simulink model "DIPCRT"  (R2015a)
settings: Solver=ode23  SolverMode=SingleTasking  StartTime=0.0  StopTime=3  FixedStep=1e-3  RelTol=1e-3
values from neighbouring files (symbols this model uses):
  deltas = 1000    [DIPCRTinit.m]
  deltav = 5000    [DIPCRTinit.m]
  ds = 1000    [DIPCRTinit.m]
  dv = 5000    [DIPCRTinit.m]
  g = [0;0;0]    [DIPCRTinit.m]
  j0 = 1    [DIPCRTinit.m]
  j1 = 10    [DIPCRTinit.m]
  j2 = 10    [DIPCRTinit.m]
  j3 = 10    [DIPCRTinit.m]
  j4 = 10    [DIPCRTinit.m]
  jv = 1    [DIPCRTinit.m]
  kappas = 2000    [DIPCRTinit.m]
  kappav = 20000    [DIPCRTinit.m]
  kpr = 500    [DIPCRTinit.m]
  kpt = 500    [DIPCRTinit.m]
  ks = 2000    [DIPCRTinit.m]
  kv = 30    [DIPCRTinit.m]
  m0 = 10    [DIPCRTinit.m]
  m1 = 10    [DIPCRTinit.m]
  m2 = 10    [DIPCRTinit.m]
  m3 = 10    [DIPCRTinit.m]
  m4 = 10    [DIPCRTinit.m]
  mv = 10    [DIPCRTinit.m]
libraries: aerolibutil x22, dspinverses x3, aerolibtransform2 x2, simulink x2
(part 1 of 2)
settings Model: CovSFcnEnable=off  Creator=Martin  LastModifiedBy=mangerer
settings OptimizationCC: BlockReduction=off  BooleanDataType=off  OptimizeBlockIOStorage=off  BufferReuse=off  GlobalBufferReuse=off  ExpressionFolding=off  LocalBlockOutputs=off
settings DebuggingCC: SaveWithParameterizedLinksMsg=none  UnderspecifiedInitializationDetection=Classic  MergeDetectMultiDrivingBlocksExec=none  SignalResolutionControl=TryResolveAllWithWarning
settings HardwareCC: TargetUnknown=on

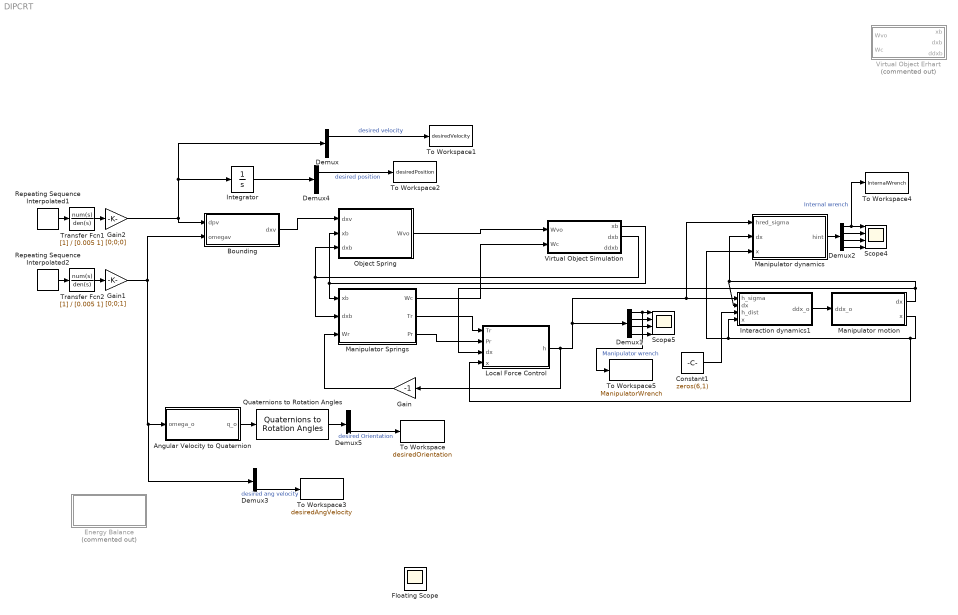
== system DIPCRT ==
  Angular Velocity to Quaternion : Subsystem
  Bounding : Subsystem
  Constant1 : Constant  Value=zeros(6,1)
  Demux{,3..5} (4 alike) : Demux  Outputs=3
  Demux1 : Demux
  Demux2 : Demux
  Energy Balance : Subsystem  Commented=on
  Floating Scope : Scope  NumInputPorts=2
      settings: Floating=on  ShowLegends=on  TimeRange=3  YMin=-0.1~-0.55  YMax=0.05~0.25
  Gain : Gain  Gain=-1
  Gain1 : Gain  Gain=[0;0;1]
  Gain2 : Gain  Gain=[0;0;0]
  Integrator : Integrator
  Interaction dynamics1 : Subsystem
  Local Force Control : Subsystem
  Manipulator Springs : Subsystem
  Manipulator dynamics : Subsystem
  Manipulator motion : Subsystem
  Object Spring : Subsystem
  Quaternions to Rotation Angles : aerolibtransform2/Quaternions to Rotation Angles  rotationOrder=XYZ
  Repeating Sequence Interpolated1 : simulink/Sources/Repeating Sequence Interpolated  OutValues="[0 0 0.225 0 0 0.225 0 0  -0.525 0 0 0.138 0 0].'"  TimeValues=[0 0.1 0.16 0.25 0.9 0.96 1.1 1.8 2 2.2 2.4 2.6 2.8 3].'  LookUpMeth=Interpolation-Use End Values  tsamp=0.001  OutMin=[]  OutMax=[]  OutDataTypeStr=double  OutputDataTypeScalingMode=double  OutDataType=fixdt(0,8)  OutScaling=2^-10
  Repeating Sequence Interpolated2 : simulink/Sources/Repeating Sequence Interpolated  OutValues="[0 0 0.225 0 0 0.225 0 0  -0.525 0 0 0.138 0 0].'"  TimeValues=[0 0.1 0.16 0.25 0.9 0.96 1.1 1.8 2 2.2 2.4 2.6 2.8 3].'  LookUpMeth=Interpolation-Use End Values  tsamp=0.001  OutMin=[]  OutMax=[]  OutDataTypeStr=double  OutputDataTypeScalingMode=double  OutDataType=fixdt(0,8)  OutScaling=2^-10
  Scope4 : Scope  NumInputPorts=4
      settings: ShowLegends=on  YMin=-0.01~-0.01~-0.04~-0.04  YMax=0.04~0.04~0.01~0.01  SaveName=ScopeData6
  Scope5 : Scope  NumInputPorts=4
      settings: ShowLegends=on  TimeRange=3  YMin=-40~-40~-40~-40  YMax=40~40~40~40  SaveName=ScopeData11
  To Workspace : ToWorkspace  VariableName=desiredOrientation  SaveFormat=Timeseries  SampleTime=-1
  To Workspace1 : ToWorkspace  VariableName=desiredVelocity  SaveFormat=Timeseries  SampleTime=-1
  To Workspace2 : ToWorkspace  VariableName=desiredPosition  SaveFormat=Timeseries  SampleTime=-1
  To Workspace3 : ToWorkspace  VariableName=desiredAngVelocity  SaveFormat=Timeseries  SampleTime=-1
  To Workspace4 : ToWorkspace  VariableName=InternalWrench  SaveFormat=Timeseries  SampleTime=-1
  To Workspace5 : ToWorkspace  VariableName=ManipulatorWrench  SaveFormat=Timeseries  SampleTime=-1
  Transfer Fcn1 : TransferFcn  Denominator=[0.005 1]
  Transfer Fcn2 : TransferFcn  Denominator=[0.005 1]
  Virtual Object Erhart : Subsystem  Commented=on
  Virtual Object Simulation : Subsystem
  wires:
  Object Spring/1(Wvo) -> Virtual Object Simulation/1(Wvo)
  Virtual Object Simulation/1(xb) -> Object Spring/2(xb), Manipulator Springs/1(xb)
  Manipulator Springs/1(Wc) -> Virtual Object Simulation/2(Wc)
  Interaction dynamics1/1(ddx_o) -> Manipulator motion/1(ddx_o)
  Constant1/1 -> Interaction dynamics1/3(h_dist)
  Manipulator motion/1(dx) -> Local Force Control/3(dx), Manipulator dynamics/2(dx), Interaction dynamics1/2(dx)
  Manipulator motion/2(x) -> Local Force Control/4(x), Manipulator dynamics/3(x), Interaction dynamics1/4(x)
  Virtual Object Simulation/2(dxb) -> Manipulator Springs/2(dxb), Object Spring/3(dxb)
  Manipulator dynamics/1(hint) -> Demux2/1
  Demux2/2 -> Scope4/2
  Demux2/4 -> Scope4/4
  Demux2/3 -> Scope4/3
  Demux2/1 -> To Workspace4/1, Scope4/1  "Internal wrench"
  Repeating Sequence Interpolated1/1 -> Transfer Fcn1/1
  Transfer Fcn1/1 -> Gain2/1
  Transfer Fcn2/1 -> Gain1/1
  Demux1/2 -> Scope5/2
  Demux1/4 -> Scope5/4
  Demux1/3 -> Scope5/3
  Demux1/1 -> To Workspace5/1, Scope5/1  "Manipulator wrench"
  Quaternions to Rotation Angles/1 -> Demux5/1
  Demux5/3 -> To Workspace/1  "desired Orientation"
  Demux3/3 -> To Workspace3/1  "desired ang velocity"
  Demux4/1 -> To Workspace2/1  "desired position"
  Demux/1 -> To Workspace1/1  "desired velocity"
  Integrator/1 -> Demux4/1
  Angular Velocity to Quaternion/1(q_o) -> Quaternions to Rotation Angles/1
  Gain1/1 -> Demux3/1, Angular Velocity to Quaternion/1(omega_o), Bounding/2(omegav)
  Gain2/1 -> Demux/1, Integrator/1, Bounding/1(dpv)
  Bounding/1(dxv) -> Object Spring/1(dxv)
  Repeating Sequence Interpolated2/1 -> Transfer Fcn2/1
  Manipulator Springs/2(Tr) -> Local Force Control/1(Tr)
  Manipulator Springs/3(Pr) -> Local Force Control/2(Pr)
  Local Force Control/1(h) -> Gain/1, Manipulator dynamics/1(hred_sigma), Interaction dynamics1/1(h_sigma), Demux1/1
  Gain/1 -> Manipulator Springs/3(Wr)

== system DIPCRT/Angular Velocity to Quaternion ==
  omega_o : Inport
  Constant : Constant  Value=0
  Gain : Gain  Gain=0.5
  Integrator : Integrator  InitialCondition=[1; 0; 0; 0]
  Mux : Mux  Inputs=2
  Quaternion Multiplication : aerolibutil/Quaternion Multiplication
  Scope : Scope
      settings: ShowLegends=on  SaveName=ScopeData9
  q_o : Outport
  wires:
  omega_o/1 -> Gain/1
  Gain/1 -> Mux/2
  Constant/1 -> Mux/1
  Quaternion Multiplication/1 -> Integrator/1
  Integrator/1 -> Quaternion Multiplication/2, q_o/1, Scope/1
  Mux/1 -> Quaternion Multiplication/1

== system DIPCRT/Bounding ==
  dpv : Inport
  omegav : Inport  Port=2
  Mux : Mux  Inputs=2
  dxv : Outport
  wires:
  dpv/1 -> Mux/1
  omegav/1 -> Mux/2
  Mux/1 -> dxv/1

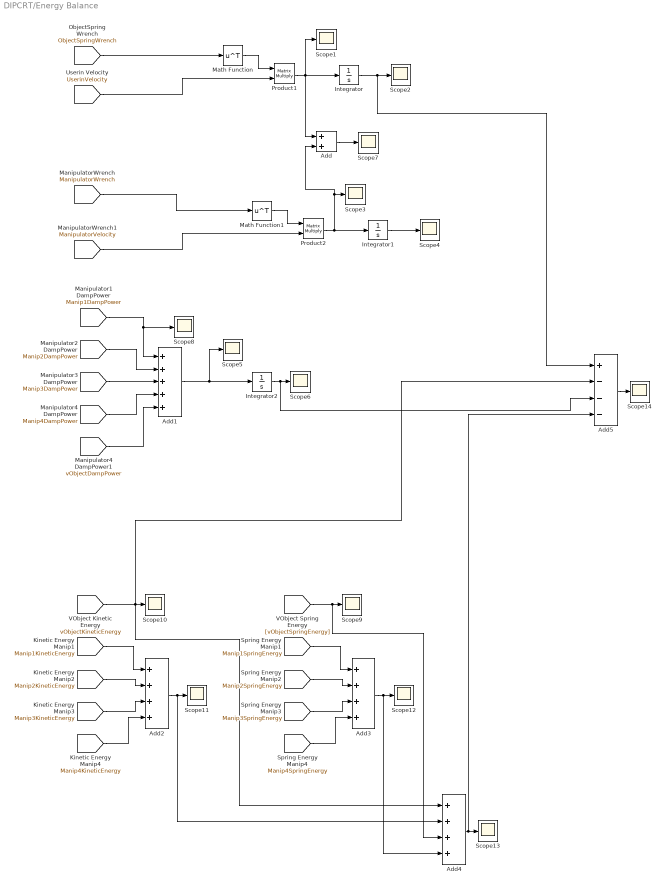
== system DIPCRT/Energy Balance ==
  Add : Sum
  Add1 : Sum  Inputs=+++++
  Add2 : Sum  Inputs=++++
  Add3 : Sum  Inputs=++++
  Add4 : Sum  Inputs=++++
  Add5 : Sum  Inputs=+---
  Integrator : Integrator
  Integrator1 : Integrator
  Integrator2 : Integrator
  Math Function : Math  Operator=transpose  SaturateOnIntegerOverflow=on
  Math Function1 : Math  Operator=transpose  SaturateOnIntegerOverflow=on
  Product1 : Product  Multiplication=Matrix(*)
  Product2 : Product  Multiplication=Matrix(*)
  Scope{1..14} (14 alike) : Scope
      Scope1 settings: YMin=0  YMax=60  SaveName=ScopeData24
      Scope10 settings: YMin=0  YMax=0.08  SaveName=ScopeData29
      Scope11 settings: YMin=0  YMax=12  SaveName=ScopeData30
      Scope12 settings: YMin=0  YMax=0.00021  SaveName=ScopeData31
      Scope13 settings: YMin=0  YMax=50  SaveName=ScopeData32
      Scope14 settings: YMin=102  YMax=108.5  SaveName=ScopeData33
      Scope2 settings: YMin=0  YMax=2100  SaveName=ScopeData18
      Scope3 settings: YMin=-60  YMax=10  SaveName=ScopeData20
      Scope4 settings: YMin=1  YMax=4.5  SaveName=ScopeData21
      Scope5 settings: YMin=-0.3  YMax=0.05  SaveName=ScopeData22
      Scope6 settings: YMin=675  YMax=1000  SaveName=ScopeData25
      Scope7 settings: YMin=-0.3  YMax=0.05  SaveName=ScopeData26
      Scope8 settings: YMin=0  YMax=3e-05  SaveName=ScopeData27
      Scope9 settings: YMin=-4.16334e-17  YMax=0.575  SaveName=ScopeData28
  wires:
  [ObjectSpringWrench] -> Math Function/1
  Product1/1 -> Add/1, Integrator/1, Scope1/1
  Math Function/1 -> Product1/1
  [UserinVelocity] -> Product1/2
  Integrator/1 -> Add5/1, Scope2/1
  Product2/1 -> Integrator1/1, Add/2, Scope3/1
  Math Function1/1 -> Product2/1
  [ManipulatorVelocity] -> Product2/2
  Integrator1/1 -> Scope4/1
  [ManipulatorWrench] -> Math Function1/1
  Add/1 -> Scope7/1
  [Manip1DampPower] -> Scope8/1, Add1/1
  [Manip2DampPower] -> Add1/2
  [Manip3DampPower] -> Add1/3
  [Manip4DampPower] -> Add1/4
  [vObjectDampPower] -> Add1/5
  Add1/1 -> Integrator2/1, Scope5/1
  [vObjectSpringEnergy] -> Add4/3, Scope9/1
  [vObjectKineticEnergy] -> Add5/2, Add4/1, Scope10/1
  [Manip1KineticEnergy] -> Add2/1
  [Manip2KineticEnergy] -> Add2/2
  [Manip3KineticEnergy] -> Add2/3
  [Manip4KineticEnergy] -> Add2/4
  Add2/1 -> Add4/2, Scope11/1
  [Manip1SpringEnergy] -> Add3/1
  [Manip2SpringEnergy] -> Add3/2
  [Manip3SpringEnergy] -> Add3/3
  [Manip4SpringEnergy] -> Add3/4
  Add3/1 -> Add4/4, Scope12/1
  Add4/1 -> Add5/4, Scope13/1
  Integrator2/1 -> Add5/3, Scope6/1
  Add5/1 -> Scope14/1

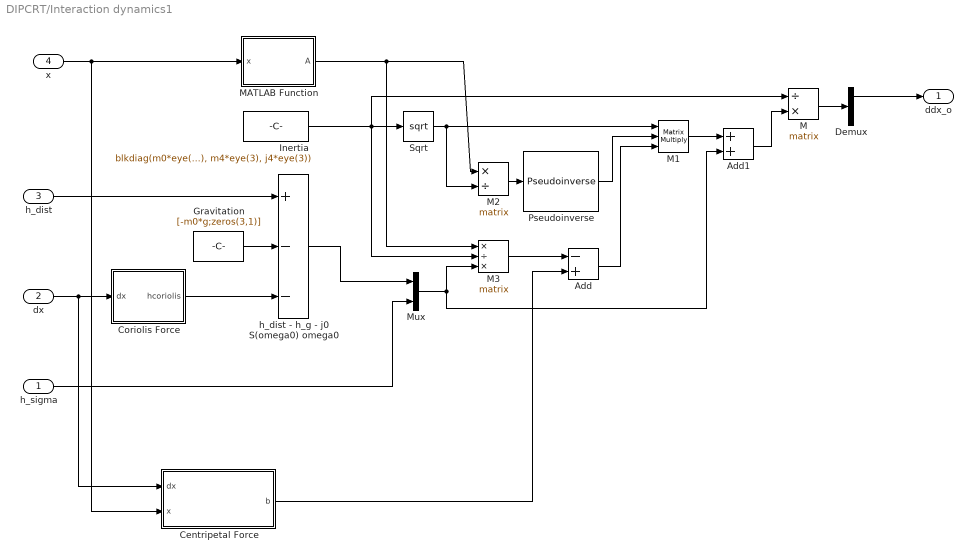
== system DIPCRT/Interaction dynamics1 ==
  h_sigma : Inport
  dx : Inport  Port=2
  h_dist : Inport  Port=3
  x : Inport  Port=4
  Add : Sum  Inputs=-+
  Add1 : Sum
  Centripetal Force : MATLAB Function  TreatAsAtomicUnit=on
  Coriolis Force : MATLAB Function  TreatAsAtomicUnit=on
  Demux : Demux  Outputs=5
  Gravitation : Constant  Value=[-m0*g;zeros(3,1)]
  Inertia : Constant  Value=blkdiag(m0*eye(3),j0*eye(3),m1*eye(3), j1*eye(3), m2*eye(3), j2*eye(3),m3*eye(3), j3*eye(3), m4*eye(3), j4*eye(3))
  M : Product  Inputs=/*  Multiplication=Matrix(*)
  M1 : Product  Inputs=***  Multiplication=Matrix(*)
  M2 : Product  Inputs=*/  Multiplication=Matrix(*)
  M3 : Product  Inputs=*/*  Multiplication=Matrix(*)
  MATLAB Function : MATLAB Function  TreatAsAtomicUnit=on
  Mux : Mux  Inputs=2
  Pseudoinverse : dspinverses/Pseudoinverse  wanterr=off
  Sqrt : Sqrt  SaturateOnIntegerOverflow=on
  "h_dist - h_g - j0 S(omega0) omega0 " : Sum  Inputs=+--
  ddx_o : Outport
  wires:
  h_dist/1 -> "h_dist - h_g - j0 S(omega0) omega0 "/1
  Gravitation/1 -> "h_dist - h_g - j0 S(omega0) omega0 "/2
  dx/1 -> Centripetal Force/1(dx), Coriolis Force/1(dx)
  Coriolis Force/1(hcoriolis) -> "h_dist - h_g - j0 S(omega0) omega0 "/3
  x/1 -> MATLAB Function/1(x), Centripetal Force/2(x)
  Inertia/1 -> M/1, M3/2, Sqrt/1
  Sqrt/1 -> M2/2, M1/1
  MATLAB Function/1(A) -> M3/1, M2/1
  M2/1 -> Pseudoinverse/1
  Pseudoinverse/1 -> M1/2
  Add/1 -> M1/3
  Centripetal Force/1(b) -> Add/2
  M3/1 -> Add/1
  Mux/1 -> Add1/2, M3/3
  "h_dist - h_g - j0 S(omega0) omega0 "/1 -> Mux/1
  h_sigma/1 -> Mux/2
  M/1 -> Demux/1
  Demux/1 -> ddx_o/1
  M1/1 -> Add1/1
  Add1/1 -> M/2

== system DIPCRT/Local Force Control ==
  Tr : Inport
  Pr : Inport  Port=2  PortDimensions=28
  dx : Inport  Port=3
  x : Inport  Port=4
  Add : Sum  Inputs=+++
  Add1 : Sum  Inputs=+-
  Derivative : Derivative
  Manipulator Inertia : Constant  Value=blkdiag(m1*eye(3), j1*eye(3), m2*eye(3), j2*eye(3), m3*eye(3), j3*eye(3), m4*eye(3), j4*eye(3))
  Manipulator kv : Constant  Value=kv*eye(24)
  Product : Product  Multiplication=Matrix(*)
  Product1 : Product  Multiplication=Matrix(*)
  Subsystem : Subsystem
  h : Outport
  wires:
  Product/1 -> h/1
  Manipulator Inertia/1 -> Product/1
  Add/1 -> Product/2
  Tr/1 -> Derivative/1, Add1/1
  dx/1 -> Add1/2
  x/1 -> Subsystem/2(x)
  Subsystem/1(hk) -> Add/1
  Add1/1 -> Product1/2
  Manipulator kv/1 -> Product1/1
  Product1/1 -> Add/2
  Pr/1 -> Subsystem/1(x_r)
  Derivative/1 -> Add/3

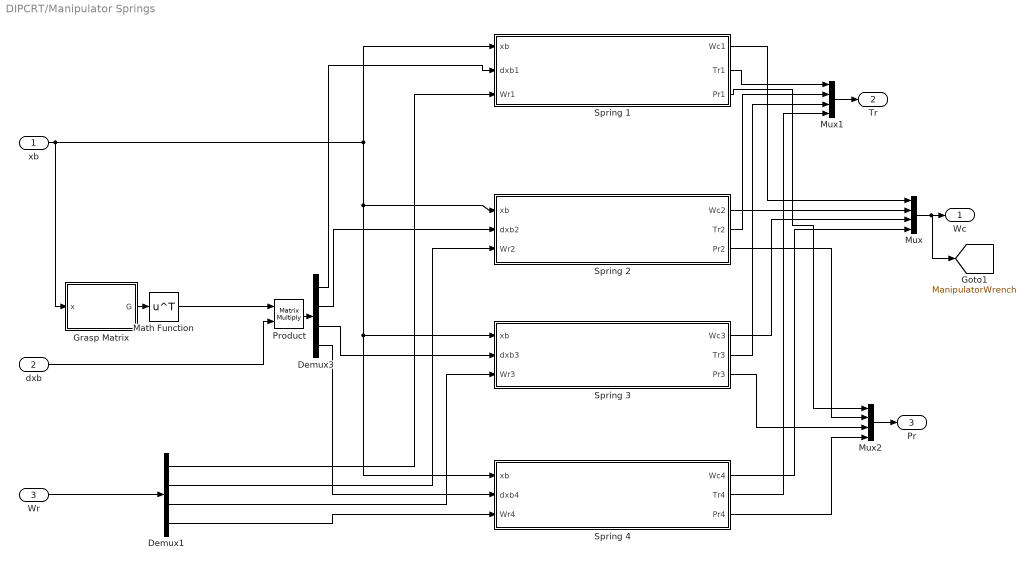
== system DIPCRT/Manipulator Springs ==
  xb : Inport
  dxb : Inport  Port=2
  Wr : Inport  Port=3
  Demux1 : Demux
  Demux3 : Demux
  Grasp Matrix : MATLAB Function  TreatAsAtomicUnit=on
  Math Function : Math  Operator=transpose  SaturateOnIntegerOverflow=on
  Mux : Mux
  Mux1 : Mux
  Mux2 : Mux
  Product : Product  Multiplication=Matrix(*)
  Spring 1 : Subsystem
  Spring 2 : Subsystem
  Spring 3 : Subsystem
  Spring 4 : Subsystem
  Wc : Outport
  Tr : Outport  Port=2
  Pr : Outport  Port=3
  tag scope: ManipulatorWrench=global
  wires:
  Spring 1/1(Wc1) -> Mux/1
  Spring 2/1(Wc2) -> Mux/2
  Mux/1 -> [ManipulatorWrench], Wc/1
  Spring 3/1(Wc3) -> Mux/3
  Spring 4/1(Wc4) -> Mux/4
  Grasp Matrix/1(G) -> Math Function/1
  Math Function/1 -> Product/1
  dxb/1 -> Product/2
  Product/1 -> Demux3/1
  xb/1 -> Spring 1/1(xb), Spring 2/1(xb), Spring 3/1(xb), Spring 4/1(xb), Grasp Matrix/1(x)
  Demux3/1 -> Spring 1/2(dxb1)
  Demux3/2 -> Spring 2/2(dxb2)
  Demux3/3 -> Spring 3/2(dxb3)
  Demux3/4 -> Spring 4/2(dxb4)
  Spring 1/2(Tr1) -> Mux1/1
  Spring 2/2(Tr2) -> Mux1/2
  Spring 3/2(Tr3) -> Mux1/3
  Spring 4/2(Tr4) -> Mux1/4
  Mux1/1 -> Tr/1
  Demux1/4 -> Spring 4/3(Wr4)
  Demux1/3 -> Spring 3/3(Wr3)
  Demux1/2 -> Spring 2/3(Wr2)
  Demux1/1 -> Spring 1/3(Wr1)
  Wr/1 -> Demux1/1
  Mux2/1 -> Pr/1
  Spring 4/3(Pr4) -> Mux2/4
  Spring 3/3(Pr3) -> Mux2/3
  Spring 2/3(Pr2) -> Mux2/2
  Spring 1/3(Pr1) -> Mux2/1

== system DIPCRT/Manipulator dynamics ==
  hred_sigma : Inport
  dx : Inport  Port=2
  x : Inport  Port=3
  A_ * M * A_' : Product  Commented=on  Inputs=*/*  Multiplication=Matrix(*)
  A_'(A_ *M *A_')^-1(b_ - A_/M*hred) : Product  Commented=on  Inputs=*/*  Multiplication=Matrix(*)
  A_/M*hred : Product  Inputs=*/*  Multiplication=Matrix(*)
  Centripal Force : MATLAB Function  TreatAsAtomicUnit=on
  Inertia : Constant  Value=blkdiag(m1*eye(3), j1*eye(3), m2*eye(3), j2*eye(3), m3*eye(3), j3*eye(3), m4*eye(3), j4*eye(3))
  Mult : Product  Inputs=***  Multiplication=Matrix(*)
  Mult1 : Product  Inputs=*/  Multiplication=Matrix(*)
  Pseudoinverse : dspinverses/Pseudoinverse  wanterr=off
  Reduced Constraint Matrix : MATLAB Function  TreatAsAtomicUnit=on
  Sqrt : Sqrt  SaturateOnIntegerOverflow=on
  Transpose : Math  Operator=transpose  SaturateOnIntegerOverflow=on
  World to Object Frame : MATLAB Function  TreatAsAtomicUnit=on
  b_ - A_/M*hred : Sum  Inputs=-+
  hint : Outport
  wires:
  Reduced Constraint Matrix/1(Ared) -> Transpose/1, A_/M*hred/1, Mult1/1
  Inertia/1 -> Sqrt/1, A_/M*hred/2
  dx/1 -> Centripal Force/2(dx)
  A_/M*hred/1 -> b_ - A_/M*hred/1
  hred_sigma/1 -> A_/M*hred/3
  World to Object Frame/1(h_int) -> hint/1
  x/1 -> Centripal Force/1(x), Reduced Constraint Matrix/1(x), World to Object Frame/2(x)
  Centripal Force/1(bred) -> b_ - A_/M*hred/2
  Mult/1 -> World to Object Frame/1(hw)
  b_ - A_/M*hred/1 -> Mult/3
  Sqrt/1 -> Mult1/2, Mult/1
  Mult1/1 -> Pseudoinverse/1
  Pseudoinverse/1 -> Mult/2

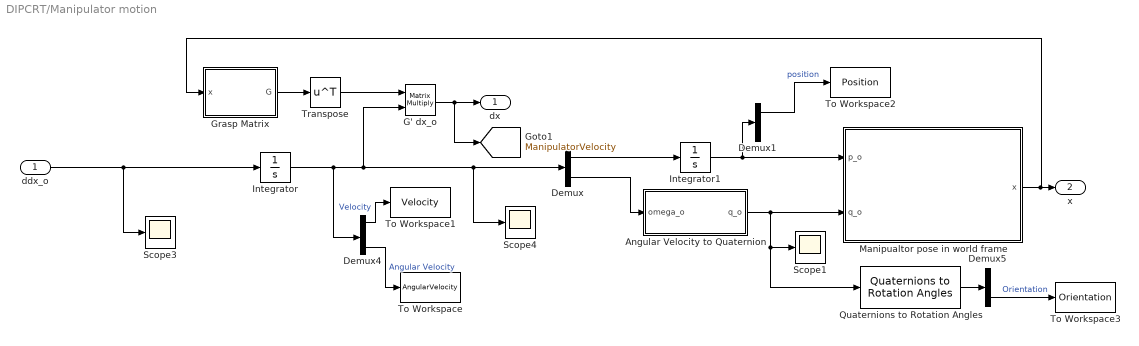
== system DIPCRT/Manipulator motion ==
  ddx_o : Inport
  Angular Velocity to Quaternion : Subsystem
  Demux : Demux  Outputs=2
  Demux1 : Demux  Outputs=3
  Demux4 : Demux  Outputs=6
  Demux5 : Demux  Outputs=3
  G' dx_o : Product  Multiplication=Matrix(*)
  Grasp Matrix : MATLAB Function  TreatAsAtomicUnit=on
  Integrator : Integrator  InitialCondition=zeros(6,1)
  Integrator1 : Integrator  InitialCondition=[0 0 0]'
  Manipualtor pose in world frame : MATLAB Function  TreatAsAtomicUnit=on
  Quaternions to Rotation Angles : aerolibtransform2/Quaternions to Rotation Angles  rotationOrder=XYZ
  Scope1 : Scope
      settings: SaveName=ScopeData13
  Scope3 : Scope
      settings: SaveName=ScopeData7
  Scope4 : Scope
      settings: SaveName=ScopeData16
  To Workspace : ToWorkspace  VariableName=AngularVelocity  SaveFormat=Timeseries  SampleTime=-1
  To Workspace1 : ToWorkspace  VariableName=Velocity  SaveFormat=Timeseries  SampleTime=-1
  To Workspace2 : ToWorkspace  VariableName=Position  SaveFormat=Timeseries  SampleTime=-1
  To Workspace3 : ToWorkspace  VariableName=Orientation  SaveFormat=Timeseries  SampleTime=-1
  Transpose : Math  Operator=transpose  SaturateOnIntegerOverflow=on
  dx : Outport
  x : Outport  Port=2
  tag scope: ManipulatorVelocity=global
  wires:
  ddx_o/1 -> Scope3/1, Integrator/1
  Integrator/1 -> Demux4/1, G' dx_o/2, Scope4/1, Demux/1
  Grasp Matrix/1(G) -> Transpose/1
  Transpose/1 -> G' dx_o/1
  G' dx_o/1 -> [ManipulatorVelocity], dx/1
  Demux/2 -> Angular Velocity to Quaternion/1(omega_o)
  Demux/1 -> Integrator1/1
  Integrator1/1 -> Demux1/1, Manipualtor pose in world frame/1(p_o)
  Manipualtor pose in world frame/1(x) -> Grasp Matrix/1(x), x/1
  Angular Velocity to Quaternion/1(q_o) -> Scope1/1, Quaternions to Rotation Angles/1, Manipualtor pose in world frame/2(q_o)
  Demux4/1 -> To Workspace1/1  "Velocity"
  Demux4/6 -> To Workspace/1  "Angular Velocity"
  Quaternions to Rotation Angles/1 -> Demux5/1
  Demux5/3 -> To Workspace3/1  "Orientation"
  Demux1/1 -> To Workspace2/1  "position"

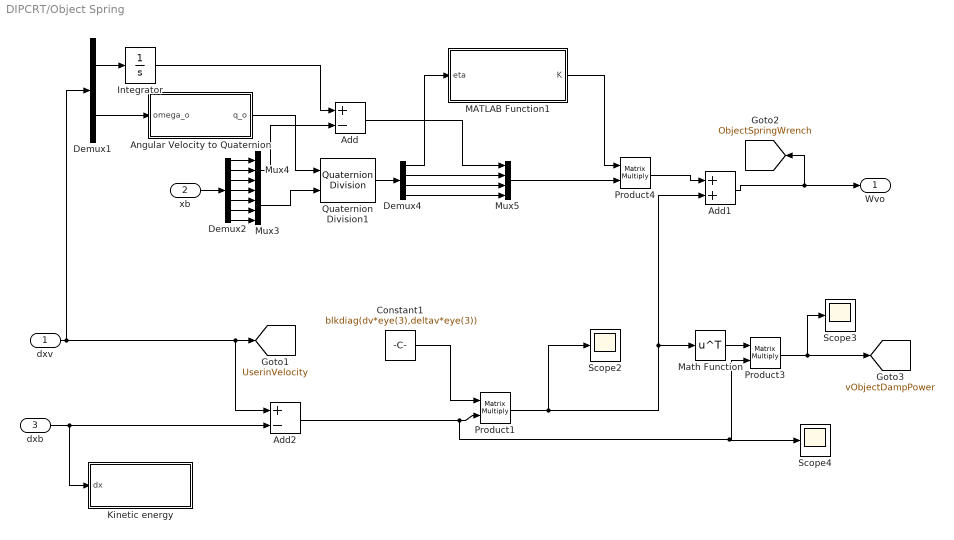
== system DIPCRT/Object Spring ==
  dxv : Inport
  xb : Inport  Port=2
  dxb : Inport  Port=3
  Add : Sum  Inputs=+-
  Add1 : Sum
  Add2 : Sum  Inputs=+-
  Angular Velocity to Quaternion : Subsystem
  Constant1 : Constant  Value=blkdiag(dv*eye(3),deltav*eye(3))
  Demux1 : Demux  Outputs=2
  Demux2 : Demux  Outputs=7
  Demux4 : Demux
  Integrator : Integrator
  Kinetic energy : Subsystem
  MATLAB Function1 : MATLAB Function  TreatAsAtomicUnit=on
  Math Function : Math  Operator=transpose  SaturateOnIntegerOverflow=on
  Mux3 : Mux
  Mux4 : Mux  Inputs=3
  Mux5 : Mux
  Product1 : Product  Multiplication=Matrix(*)
  Product3 : Product  Multiplication=Matrix(*)
  Product4 : Product  Multiplication=Matrix(*)
  Quaternion Division1 : aerolibutil/Quaternion Division
  Scope2 : Scope
      settings: YMin=-1500  YMax=6500  SaveName=ScopeData4
  Scope3 : Scope
      settings: YMin=0  YMax=8500  SaveName=ScopeData2
  Scope4 : Scope
      settings: YMin=-3.5  YMax=3  SaveName=ScopeData35
  Wvo : Outport
  tag scope: ObjectSpringWrench=global, UserinVelocity=global, vObjectDampPower=global
  wires:
  Add1/1 -> [ObjectSpringWrench], Wvo/1
  Product4/1 -> Add1/1
  Product1/1 -> Scope2/1, Math Function/1, Add1/2
  MATLAB Function1/1(K) -> Product4/1
  Demux4/1 -> MATLAB Function1/1(eta)
  Add/1 -> Mux5/1
  Demux4/2 -> Mux5/2
  Demux4/3 -> Mux5/3
  Demux4/4 -> Mux5/4
  Quaternion Division1/1 -> Demux4/1
  xb/1 -> Demux2/1
  Demux2/4 -> Mux3/1
  Demux2/5 -> Mux3/2
  Demux2/6 -> Mux3/3
  Demux2/7 -> Mux3/4
  Demux2/1 -> Mux4/1
  Demux2/2 -> Mux4/2
  Demux2/3 -> Mux4/3
  Mux4/1 -> Add/2
  Mux3/1 -> Quaternion Division1/2
  Add2/1 -> Scope4/1, Product3/2, Product1/2
  dxv/1 -> Demux1/1, [UserinVelocity], Add2/1
  dxb/1 -> Kinetic energy/1(dx), Add2/2
  Product3/1 -> Scope3/1, [vObjectDampPower]
  Math Function/1 -> Product3/1
  Mux5/1 -> Product4/2
  Demux1/1 -> Integrator/1
  Integrator/1 -> Add/1
  Demux1/2 -> Angular Velocity to Quaternion/1(omega_o)
  Angular Velocity to Quaternion/1(q_o) -> Quaternion Division1/1
  Constant1/1 -> Product1/1

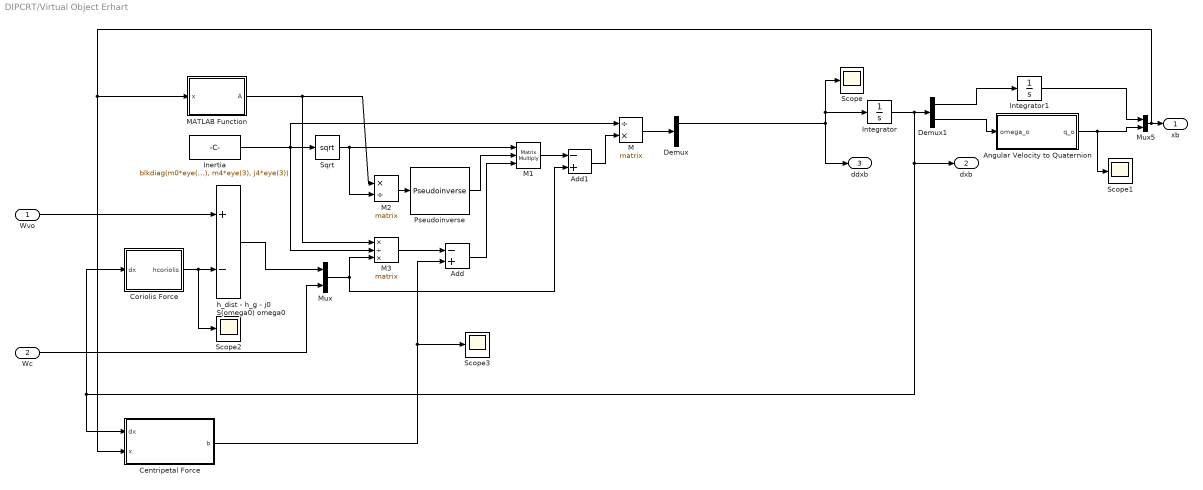
== system DIPCRT/Virtual Object Erhart ==
  Wvo : Inport
  Wc : Inport  Port=2
  Add : Sum  Inputs=-+
  Add1 : Sum  Inputs=-+
  Angular Velocity to Quaternion : Subsystem
  Centripetal Force : MATLAB Function  TreatAsAtomicUnit=on
  Coriolis Force : MATLAB Function  TreatAsAtomicUnit=on
  Demux : Demux  Outputs=5
  Demux1 : Demux  Outputs=2
  Inertia : Constant  Value=blkdiag(m0*eye(3),j0*eye(3),m1*eye(3), j1*eye(3), m2*eye(3), j2*eye(3),m3*eye(3), j3*eye(3), m4*eye(3), j4*eye(3))
  Integrator : Integrator  InitialCondition=zeros(6,1)
  Integrator1 : Integrator  InitialCondition=[0 0 0]'
  M : Product  Inputs=/*  Multiplication=Matrix(*)
  M1 : Product  Inputs=***  Multiplication=Matrix(*)
  M2 : Product  Inputs=*/  Multiplication=Matrix(*)
  M3 : Product  Inputs=*/*  Multiplication=Matrix(*)
  MATLAB Function : MATLAB Function  TreatAsAtomicUnit=on
  Mux : Mux  Inputs=2
  Mux5 : Mux  Inputs=2
  Pseudoinverse : dspinverses/Pseudoinverse  wanterr=off
  Scope{,1..3} (4 alike) : Scope
      Scope1 settings: SaveName=ScopeData8
      Scope2 settings: SaveName=ScopeData15
      Scope3 settings: YMin=-1  YMax=1  SaveName=ScopeData17
  Sqrt : Sqrt  SaturateOnIntegerOverflow=on
  "h_dist - h_g - j0 S(omega0) omega0 " : Sum  Inputs=+-
  xb : Outport
  dxb : Outport  Port=2
  ddxb : Outport  Port=3
  wires:
  Demux/1 -> Scope/1, Integrator/1, ddxb/1
  Integrator/1 -> Demux1/1, Coriolis Force/1(dx), Centripetal Force/1(dx), dxb/1
  Demux1/2 -> Angular Velocity to Quaternion/1(omega_o)
  Demux1/1 -> Integrator1/1
  Integrator1/1 -> Mux5/1
  Angular Velocity to Quaternion/1(q_o) -> Scope1/1, Mux5/2
  Wvo/1 -> "h_dist - h_g - j0 S(omega0) omega0 "/1
  Coriolis Force/1(hcoriolis) -> Scope2/1, "h_dist - h_g - j0 S(omega0) omega0 "/2
  Mux5/1 -> MATLAB Function/1(x), Centripetal Force/2(x), xb/1
  Inertia/1 -> M/1, M3/2, Sqrt/1
  Sqrt/1 -> M2/2, M1/1
  MATLAB Function/1(A) -> M3/1, M2/1
  M2/1 -> Pseudoinverse/1
  Pseudoinverse/1 -> M1/2
  Add/1 -> M1/3
  Centripetal Force/1(b) -> Scope3/1, Add/2
  M3/1 -> Add/1
  Mux/1 -> Add1/2, M3/3
  "h_dist - h_g - j0 S(omega0) omega0 "/1 -> Mux/1
  Wc/1 -> Mux/2
  M1/1 -> Add1/1
  Add1/1 -> M/2
  M/1 -> Demux/1

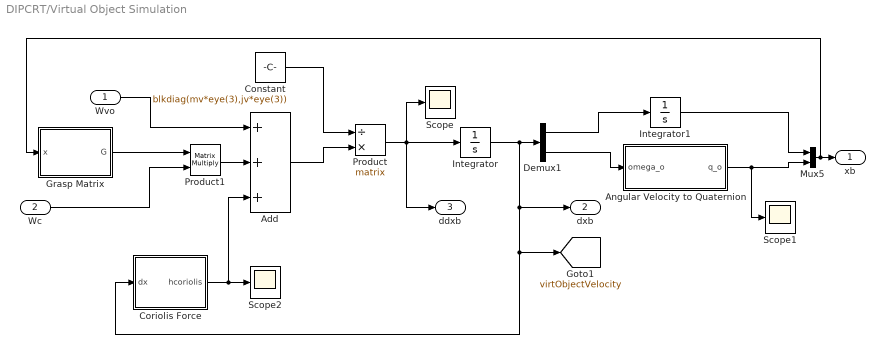
== system DIPCRT/Virtual Object Simulation ==
  Wvo : Inport
  Wc : Inport  Port=2
  Add : Sum  Inputs=+++
  Angular Velocity to Quaternion : Subsystem
  Constant : Constant  Value=blkdiag(mv*eye(3),jv*eye(3))
  Coriolis Force : MATLAB Function  TreatAsAtomicUnit=on
  Demux1 : Demux  Outputs=2
  Grasp Matrix : MATLAB Function  TreatAsAtomicUnit=on
  Integrator : Integrator  InitialCondition=zeros(6,1)
  Integrator1 : Integrator  InitialCondition=[0 0 0]'
  Mux5 : Mux  Inputs=2
  Product : Product  Inputs=/*  Multiplication=Matrix(*)
  Product1 : Product  Inputs=**  Multiplication=Matrix(*)
  Scope : Scope
  Scope1 : Scope
      settings: SaveName=ScopeData8
  Scope2 : Scope
      settings: YMin=-0.008  YMax=0.008  SaveName=ScopeData10
  xb : Outport
  dxb : Outport  Port=2
  ddxb : Outport  Port=3
  tag scope: virtObjectVelocity=global
  wires:
  Add/1 -> Product/2
  Constant/1 -> Product/1
  Product/1 -> ddxb/1, Scope/1, Integrator/1
  Integrator/1 -> Demux1/1, [virtObjectVelocity], Coriolis Force/1(dx), dxb/1
  Demux1/2 -> Angular Velocity to Quaternion/1(omega_o)
  Demux1/1 -> Integrator1/1
  Integrator1/1 -> Mux5/1
  Angular Velocity to Quaternion/1(q_o) -> Scope1/1, Mux5/2
  Mux5/1 -> Grasp Matrix/1(x), xb/1
  Wvo/1 -> Add/1
  Product1/1 -> Add/2
  Grasp Matrix/1(G) -> Product1/1
  Wc/1 -> Product1/2
  Coriolis Force/1(hcoriolis) -> Scope2/1, Add/3

== system DIPCRT/Local Force Control/Subsystem ==
  x_r : Inport
  x : Inport  Port=2
  Demux : Demux
  Demux1 : Demux
  Mux : Mux
  Subsystem : Subsystem
  Subsystem1 : Subsystem
  Subsystem2 : Subsystem
  Subsystem3 : Subsystem
  hk : Outport
  wires:
  x_r/1 -> Demux/1
  x/1 -> Demux1/1
  Demux/1 -> Subsystem/1(x_r1)
  Demux/2 -> Subsystem1/1(x_r2)
  Demux/3 -> Subsystem2/1(x_r3)
  Demux/4 -> Subsystem3/1(x_r4)
  Demux1/1 -> Subsystem/2(x1)
  Demux1/2 -> Subsystem1/2(x2)
  Demux1/3 -> Subsystem2/2(x3)
  Demux1/4 -> Subsystem3/2(x4)
  Subsystem/1(hk1) -> Mux/1
  Subsystem1/1(hk2) -> Mux/2
  Subsystem2/1(hk3) -> Mux/3
  Subsystem3/1(hk4) -> Mux/4
  Mux/1 -> hk/1

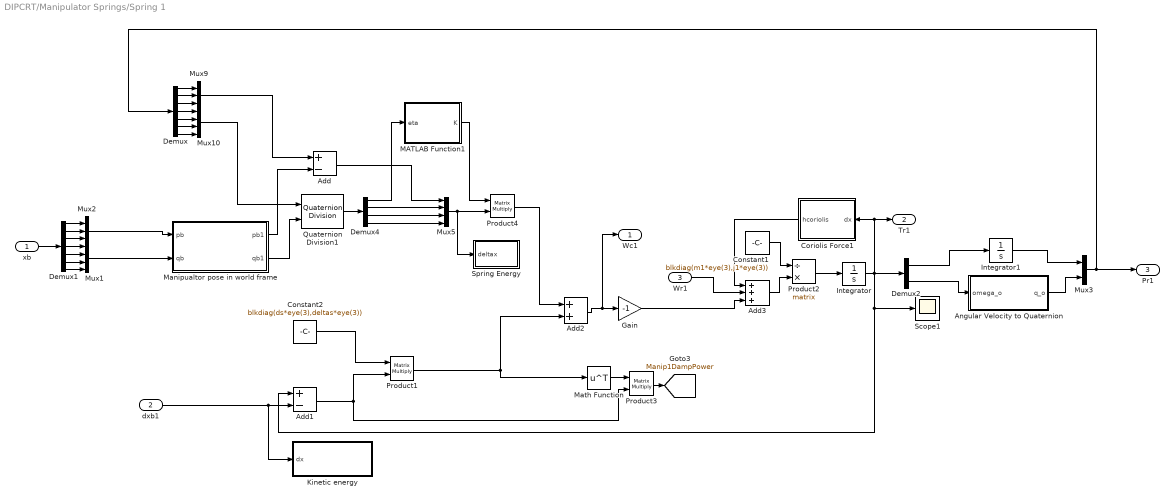
== system DIPCRT/Manipulator Springs/Spring 1 ==
  xb : Inport
  dxb1 : Inport  Port=2
  Wr1 : Inport  Port=3
  Add : Sum  Inputs=+-
  Add1 : Sum  Inputs=+-
  Add2 : Sum
  Add3 : Sum  Inputs=+++
  Angular Velocity to Quaternion : Subsystem
  Constant1 : Constant  Value=blkdiag(m1*eye(3),j1*eye(3))
  Constant2 : Constant  Value=blkdiag(ds*eye(3),deltas*eye(3))
  Coriolis Force1 : MATLAB Function  TreatAsAtomicUnit=on
  Demux : Demux  Outputs=7
  Demux1 : Demux  Outputs=7
  Demux2 : Demux  Outputs=2
  Demux4 : Demux
  Gain : Gain  Gain=-1
  Integrator : Integrator  InitialCondition=zeros(6,1)
  Integrator1 : Integrator  InitialCondition=[1 0 0]'
  Kinetic energy : Subsystem
  MATLAB Function1 : MATLAB Function  TreatAsAtomicUnit=on
  Manipualtor pose in world frame : MATLAB Function  TreatAsAtomicUnit=on
  Math Function : Math  Operator=transpose  SaturateOnIntegerOverflow=on
  Mux1 : Mux
  Mux10 : Mux
  Mux2 : Mux  Inputs=3
  Mux3 : Mux  Inputs=2
  Mux5 : Mux
  Mux9 : Mux  Inputs=3
  Product1 : Product  Multiplication=Matrix(*)
  Product2 : Product  Inputs=/*  Multiplication=Matrix(*)
  Product3 : Product  Multiplication=Matrix(*)
  Product4 : Product  Multiplication=Matrix(*)
  Quaternion Division1 : aerolibutil/Quaternion Division
  Scope1 : Scope
      settings: YMin=-1.5  YMax=0.5  SaveName=ScopeData38
  Spring Energy : Subsystem
  Wc1 : Outport
  Tr1 : Outport  Port=2
  Pr1 : Outport  Port=3  PortDimensions=7
  tag scope: Manip1DampPower=global
  wires:
  Constant2/1 -> Product1/1
  Add2/1 -> Gain/1, Wc1/1
  Demux/1 -> Mux9/1
  Demux/2 -> Mux9/2
  Demux/3 -> Mux9/3
  Demux/4 -> Mux10/1
  Demux/5 -> Mux10/2
  Demux/6 -> Mux10/3
  Demux/7 -> Mux10/4
  MATLAB Function1/1(K) -> Product4/1
  Demux4/1 -> MATLAB Function1/1(eta)
  Add/1 -> Mux5/1
  Demux4/2 -> Mux5/2
  Demux4/3 -> Mux5/3
  Demux4/4 -> Mux5/4
  Quaternion Division1/1 -> Demux4/1
  Mux5/1 -> Spring Energy/1(deltax), Product4/2
  Mux9/1 -> Add/1
  Manipualtor pose in world frame/1(pb1) -> Add/2
  Product4/1 -> Add2/1
  Mux10/1 -> Quaternion Division1/1
  Manipualtor pose in world frame/2(qb1) -> Quaternion Division1/2
  Add1/1 -> Product1/2, Product3/2
  dxb1/1 -> Kinetic energy/1(dx), Add1/2
  Demux1/1 -> Mux2/1
  Demux1/2 -> Mux2/2
  Demux1/3 -> Mux2/3
  Demux1/4 -> Mux1/1
  Demux1/5 -> Mux1/2
  Demux1/6 -> Mux1/3
  Demux1/7 -> Mux1/4
  Mux2/1 -> Manipualtor pose in world frame/1(pb)
  Mux1/1 -> Manipualtor pose in world frame/2(qb)
  xb/1 -> Demux1/1
  Product1/1 -> Add2/2, Math Function/1
  Math Function/1 -> Product3/1
  Product3/1 -> [Manip1DampPower]
  Product2/1 -> Integrator/1
  Add3/1 -> Product2/2
  Coriolis Force1/1(hcoriolis) -> Add3/1
  Demux2/2 -> Angular Velocity to Quaternion/1(omega_o)
  Demux2/1 -> Integrator1/1
  Gain/1 -> Add3/3
  Constant1/1 -> Product2/1
  Wr1/1 -> Add3/2
  Integrator/1 -> Demux2/1, Coriolis Force1/1(dx), Tr1/1, Add1/1, Scope1/1
  Angular Velocity to Quaternion/1(q_o) -> Mux3/2
  Integrator1/1 -> Mux3/1
  Mux3/1 -> Pr1/1, Demux/1

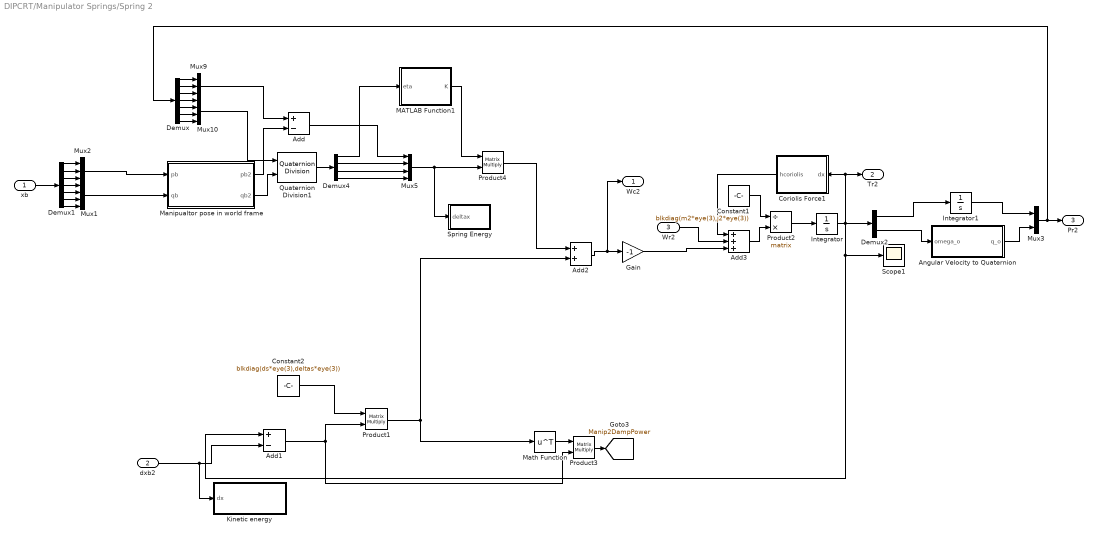
== system DIPCRT/Manipulator Springs/Spring 2 ==
  xb : Inport
  dxb2 : Inport  Port=2
  Wr2 : Inport  Port=3
  Add : Sum  Inputs=+-
  Add1 : Sum  Inputs=+-
  Add2 : Sum
  Add3 : Sum  Inputs=+++
  Angular Velocity to Quaternion : Subsystem
  Constant1 : Constant  Value=blkdiag(m2*eye(3),j2*eye(3))
  Constant2 : Constant  Value=blkdiag(ds*eye(3),deltas*eye(3))
  Coriolis Force1 : MATLAB Function  TreatAsAtomicUnit=on
  Demux : Demux  Outputs=7
  Demux1 : Demux  Outputs=7
  Demux2 : Demux  Outputs=2
  Demux4 : Demux
  Gain : Gain  Gain=-1
  Integrator : Integrator  InitialCondition=zeros(6,1)
  Integrator1 : Integrator  InitialCondition=[0 1 0]'
  Kinetic energy : Subsystem
  MATLAB Function1 : MATLAB Function  TreatAsAtomicUnit=on
  Manipualtor pose in world frame : MATLAB Function  TreatAsAtomicUnit=on
  Math Function : Math  Operator=transpose  SaturateOnIntegerOverflow=on
  Mux1 : Mux
  Mux10 : Mux
  Mux2 : Mux  Inputs=3
  Mux3 : Mux  Inputs=2
  Mux5 : Mux
  Mux9 : Mux  Inputs=3
  Product1 : Product  Multiplication=Matrix(*)
  Product2 : Product  Inputs=/*  Multiplication=Matrix(*)
  Product3 : Product  Multiplication=Matrix(*)
  Product4 : Product  Multiplication=Matrix(*)
  Quaternion Division1 : aerolibutil/Quaternion Division
  Scope1 : Scope
      settings: SaveName=ScopeData3
  Spring Energy : Subsystem
  Wc2 : Outport
  Tr2 : Outport  Port=2
  Pr2 : Outport  Port=3  PortDimensions=7
  tag scope: Manip2DampPower=global
  wires:
  Constant2/1 -> Product1/1
  Demux/1 -> Mux9/1
  Demux/2 -> Mux9/2
  Demux/3 -> Mux9/3
  Demux/4 -> Mux10/1
  Demux/5 -> Mux10/2
  Demux/6 -> Mux10/3
  Demux/7 -> Mux10/4
  MATLAB Function1/1(K) -> Product4/1
  Demux4/1 -> MATLAB Function1/1(eta)
  Add/1 -> Mux5/1
  Demux4/2 -> Mux5/2
  Demux4/3 -> Mux5/3
  Demux4/4 -> Mux5/4
  Quaternion Division1/1 -> Demux4/1
  Mux5/1 -> Spring Energy/1(deltax), Product4/2
  Mux9/1 -> Add/1
  Manipualtor pose in world frame/1(pb2) -> Add/2
  Manipualtor pose in world frame/2(qb2) -> Quaternion Division1/2
  Mux10/1 -> Quaternion Division1/1
  Add2/1 -> Wc2/1, Gain/1
  Product4/1 -> Add2/1
  dxb2/1 -> Kinetic energy/1(dx), Add1/2
  xb/1 -> Demux1/1
  Demux1/1 -> Mux2/1
  Demux1/2 -> Mux2/2
  Demux1/3 -> Mux2/3
  Demux1/4 -> Mux1/1
  Demux1/5 -> Mux1/2
  Demux1/6 -> Mux1/3
  Demux1/7 -> Mux1/4
  Mux2/1 -> Manipualtor pose in world frame/1(pb)
  Mux1/1 -> Manipualtor pose in world frame/2(qb)
  Add1/1 -> Product1/2, Product3/2
  Product1/1 -> Add2/2, Math Function/1
  Math Function/1 -> Product3/1
  Product3/1 -> [Manip2DampPower]
  Product2/1 -> Integrator/1
  Add3/1 -> Product2/2
  Coriolis Force1/1(hcoriolis) -> Add3/1
  Demux2/2 -> Angular Velocity to Quaternion/1(omega_o)
  Demux2/1 -> Integrator1/1
  Constant1/1 -> Product2/1
  Wr2/1 -> Add3/2
  Integrator/1 -> Demux2/1, Coriolis Force1/1(dx), Tr2/1, Add1/1, Scope1/1
  Angular Velocity to Quaternion/1(q_o) -> Mux3/2
  Integrator1/1 -> Mux3/1
  Gain/1 -> Add3/3
  Mux3/1 -> Pr2/1, Demux/1

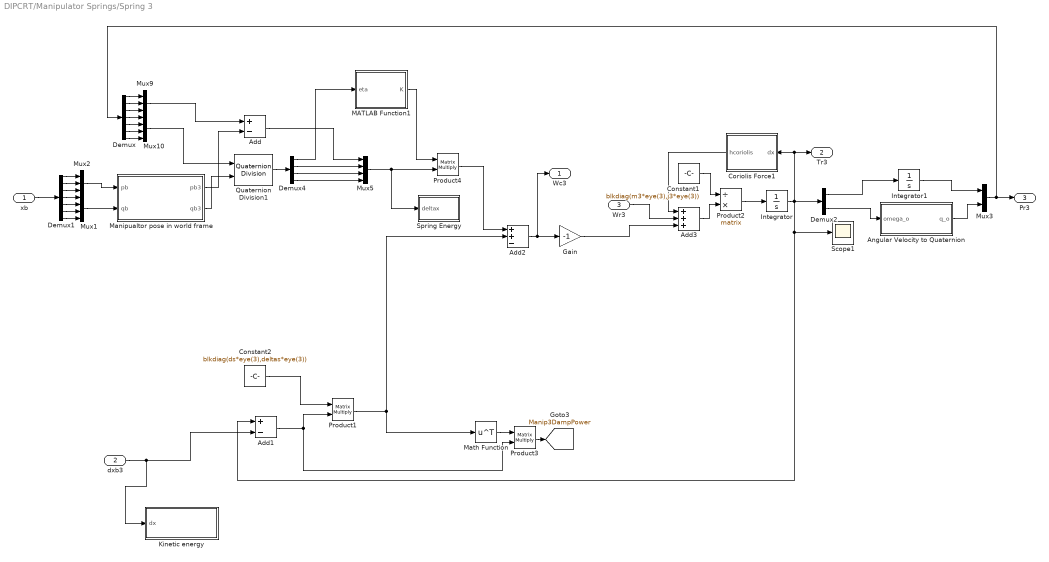
== system DIPCRT/Manipulator Springs/Spring 3 ==
  xb : Inport
  dxb3 : Inport  Port=2
  Wr3 : Inport  Port=3
  Add : Sum  Inputs=+-
  Add1 : Sum  Inputs=+-
  Add2 : Sum  Inputs=++-
  Add3 : Sum  Inputs=+++
  Angular Velocity to Quaternion : Subsystem
  Constant1 : Constant  Value=blkdiag(m3*eye(3),j3*eye(3))
  Constant2 : Constant  Value=blkdiag(ds*eye(3),deltas*eye(3))
  Coriolis Force1 : MATLAB Function  TreatAsAtomicUnit=on
  Demux : Demux  Outputs=7
  Demux1 : Demux  Outputs=7
  Demux2 : Demux  Outputs=2
  Demux4 : Demux
  Gain : Gain  Gain=-1
  Integrator : Integrator  InitialCondition=zeros(6,1)
  Integrator1 : Integrator  InitialCondition=[-1 0 0]'
  Kinetic energy : Subsystem
  MATLAB Function1 : MATLAB Function  TreatAsAtomicUnit=on
  Manipualtor pose in world frame : MATLAB Function  TreatAsAtomicUnit=on
  Math Function : Math  Operator=transpose  SaturateOnIntegerOverflow=on
  Mux1 : Mux
  Mux10 : Mux
  Mux2 : Mux  Inputs=3
  Mux3 : Mux  Inputs=2
  Mux5 : Mux
  Mux9 : Mux  Inputs=3
  Product1 : Product  Multiplication=Matrix(*)
  Product2 : Product  Inputs=/*  Multiplication=Matrix(*)
  Product3 : Product  Multiplication=Matrix(*)
  Product4 : Product  Multiplication=Matrix(*)
  Quaternion Division1 : aerolibutil/Quaternion Division
  Scope1 : Scope
      settings: SaveName=ScopeData36
  Spring Energy : Subsystem
  Wc3 : Outport
  Tr3 : Outport  Port=2
  Pr3 : Outport  Port=3  PortDimensions=7
  tag scope: Manip3DampPower=global
  wires:
  Constant2/1 -> Product1/1
  Add2/1 -> Gain/1, Wc3/1
  Demux/1 -> Mux9/1
  Demux/2 -> Mux9/2
  Demux/3 -> Mux9/3
  Demux/4 -> Mux10/1
  Demux/5 -> Mux10/2
  Demux/6 -> Mux10/3
  Demux/7 -> Mux10/4
  MATLAB Function1/1(K) -> Product4/1
  Demux4/1 -> MATLAB Function1/1(eta)
  Add/1 -> Mux5/1
  Demux4/2 -> Mux5/2
  Demux4/3 -> Mux5/3
  Demux4/4 -> Mux5/4
  Quaternion Division1/1 -> Demux4/1
  Mux5/1 -> Spring Energy/1(deltax), Product4/2
  Product4/1 -> Add2/1
  Mux9/1 -> Add/1
  Manipualtor pose in world frame/1(pb3) -> Add/2
  Mux10/1 -> Quaternion Division1/1
  Manipualtor pose in world frame/2(qb3) -> Quaternion Division1/2
  dxb3/1 -> Add1/2, Kinetic energy/1(dx)
  xb/1 -> Demux1/1
  Demux1/1 -> Mux2/1
  Demux1/2 -> Mux2/2
  Demux1/3 -> Mux2/3
  Demux1/4 -> Mux1/1
  Demux1/5 -> Mux1/2
  Demux1/6 -> Mux1/3
  Demux1/7 -> Mux1/4
  Mux2/1 -> Manipualtor pose in world frame/1(pb)
  Mux1/1 -> Manipualtor pose in world frame/2(qb)
  Add1/1 -> Product1/2, Product3/2
  Product1/1 -> Add2/2, Math Function/1
  Math Function/1 -> Product3/1
  Product3/1 -> [Manip3DampPower]
  Product2/1 -> Integrator/1
  Add3/1 -> Product2/2
  Coriolis Force1/1(hcoriolis) -> Add3/1
  Demux2/2 -> Angular Velocity to Quaternion/1(omega_o)
  Demux2/1 -> Integrator1/1
  Constant1/1 -> Product2/1
  Wr3/1 -> Add3/2
  Integrator/1 -> Demux2/1, Coriolis Force1/1(dx), Tr3/1, Add1/1, Scope1/1
  Angular Velocity to Quaternion/1(q_o) -> Mux3/2
  Integrator1/1 -> Mux3/1
  Gain/1 -> Add3/3
  Mux3/1 -> Pr3/1, Demux/1

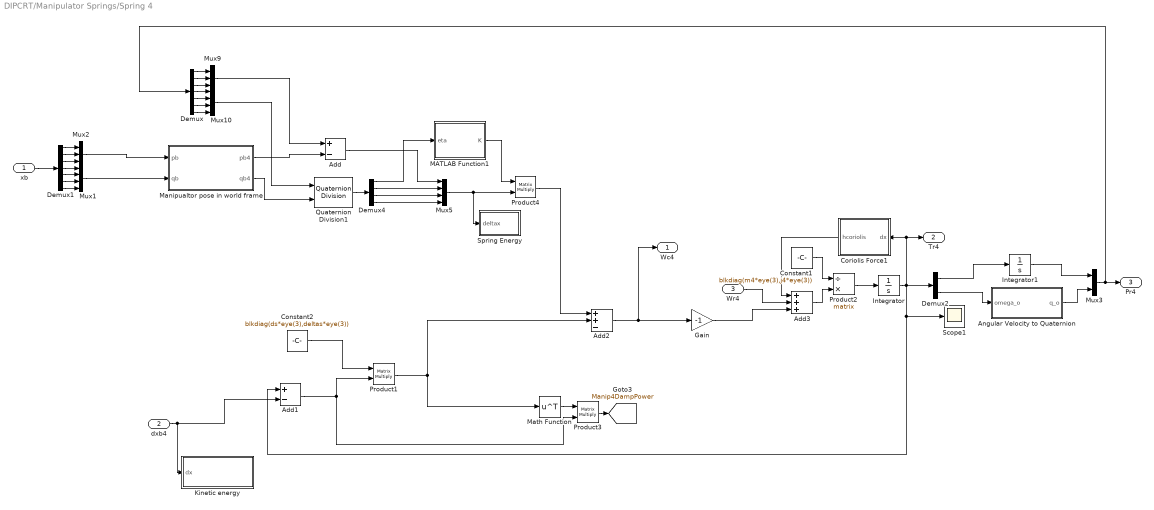
== system DIPCRT/Manipulator Springs/Spring 4 ==
  xb : Inport
  dxb4 : Inport  Port=2
  Wr4 : Inport  Port=3
  Add : Sum  Inputs=+-
  Add1 : Sum  Inputs=+-
  Add2 : Sum  Inputs=++-
  Add3 : Sum  Inputs=+++
  Angular Velocity to Quaternion : Subsystem
  Constant1 : Constant  Value=blkdiag(m4*eye(3),j4*eye(3))
  Constant2 : Constant  Value=blkdiag(ds*eye(3),deltas*eye(3))
  Coriolis Force1 : MATLAB Function  TreatAsAtomicUnit=on
  Demux : Demux  Outputs=7
  Demux1 : Demux  Outputs=7
  Demux2 : Demux  Outputs=2
  Demux4 : Demux
  Gain : Gain  Gain=-1
  Integrator : Integrator  InitialCondition=zeros(6,1)
  Integrator1 : Integrator  InitialCondition=[0 -1 0]'
  Kinetic energy : Subsystem
  MATLAB Function1 : MATLAB Function  TreatAsAtomicUnit=on
  Manipualtor pose in world frame : MATLAB Function  TreatAsAtomicUnit=on
  Math Function : Math  Operator=transpose  SaturateOnIntegerOverflow=on
  Mux1 : Mux
  Mux10 : Mux
  Mux2 : Mux  Inputs=3
  Mux3 : Mux  Inputs=2
  Mux5 : Mux
  Mux9 : Mux  Inputs=3
  Product1 : Product  Multiplication=Matrix(*)
  Product2 : Product  Inputs=/*  Multiplication=Matrix(*)
  Product3 : Product  Multiplication=Matrix(*)
  Product4 : Product  Multiplication=Matrix(*)
  Quaternion Division1 : aerolibutil/Quaternion Division
  Scope1 : Scope
      settings: SaveName=ScopeData37
  Spring Energy : Subsystem
  Wc4 : Outport
  Tr4 : Outport  Port=2
  Pr4 : Outport  Port=3  PortDimensions=7
  tag scope: Manip4DampPower=global
  wires:
  Constant2/1 -> Product1/1
  Add2/1 -> Gain/1, Wc4/1
  Demux/1 -> Mux9/1
  Demux/2 -> Mux9/2
  Demux/3 -> Mux9/3
  Demux/4 -> Mux10/1
  Demux/5 -> Mux10/2
  Demux/6 -> Mux10/3
  Demux/7 -> Mux10/4
  Demux4/2 -> Mux5/2
  Demux4/3 -> Mux5/3
  Demux4/4 -> Mux5/4
  Quaternion Division1/1 -> Demux4/1
  Mux5/1 -> Spring Energy/1(deltax), Product4/2
  MATLAB Function1/1(K) -> Product4/1
  Demux4/1 -> MATLAB Function1/1(eta)
  Add/1 -> Mux5/1
  Mux9/1 -> Add/1
  Manipualtor pose in world frame/1(pb4) -> Add/2
  Mux10/1 -> Quaternion Division1/1
  Manipualtor pose in world frame/2(qb4) -> Quaternion Division1/2
  Product4/1 -> Add2/1
  dxb4/1 -> Kinetic energy/1(dx), Add1/2
  xb/1 -> Demux1/1
  Demux1/1 -> Mux2/1
  Demux1/2 -> Mux2/2
  Demux1/3 -> Mux2/3
  Demux1/4 -> Mux1/1
  Demux1/5 -> Mux1/2
  Demux1/6 -> Mux1/3
  Demux1/7 -> Mux1/4
  Mux2/1 -> Manipualtor pose in world frame/1(pb)
  Mux1/1 -> Manipualtor pose in world frame/2(qb)
  Add1/1 -> Product1/2, Product3/2
  Product1/1 -> Add2/2, Math Function/1
  Math Function/1 -> Product3/1
  Product3/1 -> [Manip4DampPower]
  Product2/1 -> Integrator/1
  Add3/1 -> Product2/2
  Coriolis Force1/1(hcoriolis) -> Add3/1
  Demux2/2 -> Angular Velocity to Quaternion/1(omega_o)
  Demux2/1 -> Integrator1/1
  Constant1/1 -> Product2/1
  Wr4/1 -> Add3/2
  Integrator/1 -> Demux2/1, Coriolis Force1/1(dx), Tr4/1, Add1/1, Scope1/1
  Angular Velocity to Quaternion/1(q_o) -> Mux3/2
  Integrator1/1 -> Mux3/1
  Gain/1 -> Add3/3
  Mux3/1 -> Pr4/1, Demux/1

== system DIPCRT/Manipulator motion/Angular Velocity to Quaternion ==
  omega_o : Inport
  Constant : Constant  Value=0
  Gain : Gain  Gain=0.5
  Integrator : Integrator  InitialCondition=[1; 0; 0; 0]
  Mux : Mux  Inputs=2
  Quaternion Multiplication : aerolibutil/Quaternion Multiplication
  Scope : Scope
      settings: ShowLegends=on  SaveName=ScopeData9
  q_o : Outport
  wires:
  omega_o/1 -> Gain/1
  Gain/1 -> Mux/2
  Constant/1 -> Mux/1
  Quaternion Multiplication/1 -> Integrator/1
  Integrator/1 -> Quaternion Multiplication/2, q_o/1, Scope/1
  Mux/1 -> Quaternion Multiplication/1

== system DIPCRT/Object Spring/Angular Velocity to Quaternion ==
  omega_o : Inport
  Constant : Constant  Value=0
  Gain : Gain  Gain=0.5
  Integrator : Integrator  InitialCondition=[1; 0; 0; 0]
  Mux : Mux  Inputs=2
  Quaternion Multiplication : aerolibutil/Quaternion Multiplication
  Scope : Scope
      settings: ShowLegends=on  SaveName=ScopeData9
  q_o : Outport
  wires:
  omega_o/1 -> Gain/1
  Gain/1 -> Mux/2
  Constant/1 -> Mux/1
  Quaternion Multiplication/1 -> Integrator/1
  Integrator/1 -> Quaternion Multiplication/2, q_o/1, Scope/1
  Mux/1 -> Quaternion Multiplication/1

== system DIPCRT/Object Spring/Kinetic energy ==
  dx : Inport
  Constant : Constant  Value=blkdiag(0.5*mv*eye(3),0.5*jv*eye(3))
  Math Function : Math  Operator=transpose  SaturateOnIntegerOverflow=on
  Product : Product  Inputs=3  Multiplication=Matrix(*)
  tag scope: vObjectKineticEnergy=global
  wires:
  dx/1 -> Product/3, Math Function/1
  Math Function/1 -> Product/1
  Constant/1 -> Product/2
  Product/1 -> [vObjectKineticEnergy]

== system DIPCRT/Virtual Object Erhart/Angular Velocity to Quaternion ==
  omega_o : Inport
  Constant : Constant  Value=0
  Gain : Gain  Gain=0.5
  Integrator : Integrator  InitialCondition=[1; 0; 0; 0]
  Mux : Mux  Inputs=2
  Quaternion Multiplication : aerolibutil/Quaternion Multiplication
  Scope : Scope
      settings: ShowLegends=on  SaveName=ScopeData9
  q_o : Outport
  wires:
  omega_o/1 -> Gain/1
  Gain/1 -> Mux/2
  Constant/1 -> Mux/1
  Quaternion Multiplication/1 -> Integrator/1
  Integrator/1 -> Quaternion Multiplication/2, q_o/1, Scope/1
  Mux/1 -> Quaternion Multiplication/1

== system DIPCRT/Virtual Object Simulation/Angular Velocity to Quaternion ==
  omega_o : Inport
  Constant : Constant  Value=0
  Gain : Gain  Gain=0.5
  Integrator : Integrator  InitialCondition=[1; 0; 0; 0]
  Mux : Mux  Inputs=2
  Quaternion Multiplication : aerolibutil/Quaternion Multiplication
  Scope : Scope
      settings: ShowLegends=on  SaveName=ScopeData9
  q_o : Outport
  wires:
  omega_o/1 -> Gain/1
  Gain/1 -> Mux/2
  Constant/1 -> Mux/1
  Quaternion Multiplication/1 -> Integrator/1
  Integrator/1 -> Quaternion Multiplication/2, q_o/1, Scope/1
  Mux/1 -> Quaternion Multiplication/1

== system DIPCRT/Local Force Control/Subsystem/Subsystem ==
  x_r1 : Inport
  x1 : Inport  Port=2
  Add1 : Sum  Inputs=+-
  Demux1 : Demux
  Demux2 : Demux  Outputs=7
  Demux3 : Demux  Outputs=7
  Mux : Mux
  Mux1 : Mux  Inputs=3
  Mux2 : Mux
  Mux3 : Mux  Inputs=3
  Mux4 : Mux
  Prod : Product  Multiplication=Matrix(*)
  Quaternion Division1 : aerolibutil/Quaternion Division
  k1; 2kappa1*eta1 : MATLAB Function  TreatAsAtomicUnit=on
  hk1 : Outport
  wires:
  k1; 2kappa1*eta1/1(K) -> Prod/1
  Demux1/1 -> k1; 2kappa1*eta1/1(eta1)
  Mux/1 -> Prod/2
  Quaternion Division1/1 -> Demux1/1
  Prod/1 -> hk1/1
  Demux1/4 -> Mux/4
  Demux1/3 -> Mux/3
  Demux1/2 -> Mux/2
  Demux2/1 -> Mux1/1
  Demux2/2 -> Mux1/2
  Demux2/3 -> Mux1/3
  Demux2/4 -> Mux2/1
  Demux2/5 -> Mux2/2
  Demux2/6 -> Mux2/3
  Demux2/7 -> Mux2/4
  x_r1/1 -> Demux2/1
  Demux3/1 -> Mux3/1
  Demux3/2 -> Mux3/2
  Demux3/3 -> Mux3/3
  Demux3/4 -> Mux4/1
  Demux3/5 -> Mux4/2
  Demux3/6 -> Mux4/3
  Demux3/7 -> Mux4/4
  x1/1 -> Demux3/1
  Mux1/1 -> Add1/1
  Mux3/1 -> Add1/2
  Mux2/1 -> Quaternion Division1/1
  Mux4/1 -> Quaternion Division1/2
  Add1/1 -> Mux/1

== system DIPCRT/Local Force Control/Subsystem/Subsystem1 ==
  x_r2 : Inport
  x2 : Inport  Port=2
  Add2 : Sum  Inputs=+-
  Demux4 : Demux
  Demux5 : Demux  Outputs=7
  Demux6 : Demux  Outputs=7
  Mux5 : Mux
  Mux6 : Mux  Inputs=3
  Mux7 : Mux
  Mux8 : Mux  Inputs=3
  Mux9 : Mux
  Prod1 : Product  Multiplication=Matrix(*)
  Quaternion Division2 : aerolibutil/Quaternion Division
  k1; 2kappa1*eta2 : MATLAB Function  TreatAsAtomicUnit=on
  hk2 : Outport
  wires:
  Demux5/6 -> Mux7/3
  Demux6/1 -> Mux8/1
  x_r2/1 -> Demux5/1
  Demux6/3 -> Mux8/3
  Demux6/2 -> Mux8/2
  Demux6/5 -> Mux9/2
  Demux6/4 -> Mux9/1
  Demux6/7 -> Mux9/4
  Demux6/6 -> Mux9/3
  Mux6/1 -> Add2/1
  x2/1 -> Demux6/1
  Mux7/1 -> Quaternion Division2/1
  Mux8/1 -> Add2/2
  Add2/1 -> Mux5/1
  Mux9/1 -> Quaternion Division2/2
  k1; 2kappa1*eta2/1(K) -> Prod1/1
  Demux4/1 -> k1; 2kappa1*eta2/1(eta2)
  Mux5/1 -> Prod1/2
  Quaternion Division2/1 -> Demux4/1
  Prod1/1 -> hk2/1
  Demux4/4 -> Mux5/4
  Demux4/3 -> Mux5/3
  Demux4/2 -> Mux5/2
  Demux5/1 -> Mux6/1
  Demux5/2 -> Mux6/2
  Demux5/3 -> Mux6/3
  Demux5/4 -> Mux7/1
  Demux5/7 -> Mux7/4
  Demux5/5 -> Mux7/2

== system DIPCRT/Local Force Control/Subsystem/Subsystem2 ==
  x_r3 : Inport
  x3 : Inport  Port=2
  Add3 : Sum  Inputs=+-
  Demux7 : Demux
  Demux8 : Demux  Outputs=7
  Demux9 : Demux  Outputs=7
  Mux10 : Mux
  Mux11 : Mux  Inputs=3
  Mux12 : Mux
  Mux13 : Mux  Inputs=3
  Mux14 : Mux
  Prod2 : Product  Multiplication=Matrix(*)
  Quaternion Division3 : aerolibutil/Quaternion Division
  k1; 2kappa1*eta3 : MATLAB Function  TreatAsAtomicUnit=on
  hk3 : Outport
  wires:
  Demux7/1 -> k1; 2kappa1*eta3/1(eta3)
  Prod2/1 -> hk3/1
  Demux8/1 -> Mux11/1
  Demux7/3 -> Mux10/3
  Demux7/2 -> Mux10/2
  Quaternion Division3/1 -> Demux7/1
  Mux10/1 -> Prod2/2
  Demux7/4 -> Mux10/4
  Demux8/7 -> Mux12/4
  Demux9/2 -> Mux13/2
  Demux9/1 -> Mux13/1
  Demux8/2 -> Mux11/2
  Demux8/3 -> Mux11/3
  Demux8/4 -> Mux12/1
  x_r3/1 -> Demux8/1
  Demux8/5 -> Mux12/2
  Demux8/6 -> Mux12/3
  Demux9/5 -> Mux14/2
  Demux9/7 -> Mux14/4
  Mux11/1 -> Add3/1
  k1; 2kappa1*eta3/1(K) -> Prod2/1
  x3/1 -> Demux9/1
  Add3/1 -> Mux10/1
  Mux13/1 -> Add3/2
  Mux12/1 -> Quaternion Division3/1
  Mux14/1 -> Quaternion Division3/2
  Demux9/4 -> Mux14/1
  Demux9/3 -> Mux13/3
  Demux9/6 -> Mux14/3

== system DIPCRT/Local Force Control/Subsystem/Subsystem3 ==
  x_r4 : Inport
  x4 : Inport  Port=2
  Add4 : Sum  Inputs=+-
  Demux10 : Demux
  Demux11 : Demux  Outputs=7
  Demux12 : Demux  Outputs=7
  Mux15 : Mux
  Mux16 : Mux  Inputs=3
  Mux17 : Mux
  Mux18 : Mux  Inputs=3
  Mux19 : Mux
  Prod3 : Product  Multiplication=Matrix(*)
  Quaternion Division4 : aerolibutil/Quaternion Division
  k1; 2kappa1*eta4 : MATLAB Function  TreatAsAtomicUnit=on
  hk4 : Outport
  wires:
  k1; 2kappa1*eta4/1(K) -> Prod3/1
  Demux10/1 -> k1; 2kappa1*eta4/1(eta4)
  Mux15/1 -> Prod3/2
  Quaternion Division4/1 -> Demux10/1
  Prod3/1 -> hk4/1
  Demux10/4 -> Mux15/4
  Demux10/3 -> Mux15/3
  Demux10/2 -> Mux15/2
  Demux11/1 -> Mux16/1
  Demux11/2 -> Mux16/2
  Demux11/3 -> Mux16/3
  Demux11/4 -> Mux17/1
  Demux11/5 -> Mux17/2
  Demux11/6 -> Mux17/3
  Demux11/7 -> Mux17/4
  x_r4/1 -> Demux11/1
  Demux12/1 -> Mux18/1
  Demux12/2 -> Mux18/2
  Demux12/3 -> Mux18/3
  Demux12/4 -> Mux19/1
  Demux12/5 -> Mux19/2
  Demux12/6 -> Mux19/3
  Demux12/7 -> Mux19/4
  x4/1 -> Demux12/1
  Mux16/1 -> Add4/1
  Mux18/1 -> Add4/2
  Mux17/1 -> Quaternion Division4/1
  Mux19/1 -> Quaternion Division4/2
  Add4/1 -> Mux15/1

== system DIPCRT/Manipulator Springs/Spring 1/Angular Velocity to Quaternion ==
  omega_o : Inport
  Constant : Constant  Value=0
  Gain : Gain  Gain=0.5
  Integrator : Integrator  InitialCondition=[1; 0; 0; 0]
  Mux : Mux  Inputs=2
  Quaternion Multiplication : aerolibutil/Quaternion Multiplication
  Quaternion Normalize : aerolibutil/Quaternion Normalize
  q_o : Outport
  wires:
  omega_o/1 -> Gain/1
  Gain/1 -> Mux/2
  Constant/1 -> Mux/1
  Quaternion Multiplication/1 -> Integrator/1
  Integrator/1 -> Quaternion Normalize/1
  Mux/1 -> Quaternion Multiplication/1
  Quaternion Normalize/1 -> Quaternion Multiplication/2, q_o/1

== system DIPCRT/Manipulator Springs/Spring 1/Kinetic energy ==
  dx : Inport
  Constant : Constant  Value=blkdiag(0.5*m1*eye(3),0.5*j1*eye(3))
  Math Function : Math  Operator=transpose  SaturateOnIntegerOverflow=on
  Product : Product  Inputs=3  Multiplication=Matrix(*)
  tag scope: Manip1KineticEnergy=global
  wires:
  dx/1 -> Product/3, Math Function/1
  Math Function/1 -> Product/1
  Constant/1 -> Product/2
  Product/1 -> [Manip1KineticEnergy]

== system DIPCRT/Manipulator Springs/Spring 1/Spring Energy ==
  deltax : Inport
  Constant : Constant  Value=blkdiag(0.5*ks*eye(3),2*kappas*eye(3))
  Math Function : Math  Operator=transpose  SaturateOnIntegerOverflow=on
  Product : Product  Inputs=3  Multiplication=Matrix(*)
  tag scope: Manip1SpringEnergy=global
  wires:
  deltax/1 -> Product/3, Math Function/1
  Math Function/1 -> Product/1
  Constant/1 -> Product/2
  Product/1 -> [Manip1SpringEnergy]

== system DIPCRT/Manipulator Springs/Spring 2/Angular Velocity to Quaternion ==
  omega_o : Inport
  Constant : Constant  Value=0
  Gain : Gain  Gain=0.5
  Integrator : Integrator  InitialCondition=[1; 0; 0; 0]
  Mux : Mux  Inputs=2
  Quaternion Multiplication : aerolibutil/Quaternion Multiplication
  Quaternion Normalize : aerolibutil/Quaternion Normalize
  q_o : Outport
  wires:
  omega_o/1 -> Gain/1
  Gain/1 -> Mux/2
  Constant/1 -> Mux/1
  Quaternion Multiplication/1 -> Integrator/1
  Integrator/1 -> Quaternion Normalize/1
  Mux/1 -> Quaternion Multiplication/1
  Quaternion Normalize/1 -> Quaternion Multiplication/2, q_o/1

== system DIPCRT/Manipulator Springs/Spring 2/Kinetic energy ==
  dx : Inport
  Constant : Constant  Value=blkdiag(0.5*m2*eye(3),0.5*j2*eye(3))
  Math Function : Math  Operator=transpose  SaturateOnIntegerOverflow=on
  Product : Product  Inputs=3  Multiplication=Matrix(*)
  tag scope: Manip2KineticEnergy=global
  wires:
  dx/1 -> Product/3, Math Function/1
  Math Function/1 -> Product/1
  Constant/1 -> Product/2
  Product/1 -> [Manip2KineticEnergy]

== system DIPCRT/Manipulator Springs/Spring 2/Spring Energy ==
  deltax : Inport
  Constant : Constant  Value=blkdiag(0.5*ks*eye(3),2*kappas*eye(3))
  Math Function : Math  Operator=transpose  SaturateOnIntegerOverflow=on
  Product : Product  Inputs=3  Multiplication=Matrix(*)
  tag scope: Manip2SpringEnergy=global
  wires:
  deltax/1 -> Product/3, Math Function/1
  Math Function/1 -> Product/1
  Constant/1 -> Product/2
  Product/1 -> [Manip2SpringEnergy]

== system DIPCRT/Manipulator Springs/Spring 3/Angular Velocity to Quaternion ==
  omega_o : Inport
  Constant : Constant  Value=0
  Gain : Gain  Gain=0.5
  Integrator : Integrator  InitialCondition=[1; 0; 0; 0]
  Mux : Mux  Inputs=2
  Quaternion Multiplication : aerolibutil/Quaternion Multiplication
  Quaternion Normalize : aerolibutil/Quaternion Normalize
  q_o : Outport
  wires:
  omega_o/1 -> Gain/1
  Gain/1 -> Mux/2
  Constant/1 -> Mux/1
  Quaternion Multiplication/1 -> Integrator/1
  Integrator/1 -> Quaternion Normalize/1
  Mux/1 -> Quaternion Multiplication/1
  Quaternion Normalize/1 -> Quaternion Multiplication/2, q_o/1

== system DIPCRT/Manipulator Springs/Spring 3/Kinetic energy ==
  dx : Inport
  Constant : Constant  Value=blkdiag(0.5*m3*eye(3),0.5*j3*eye(3))
  Math Function : Math  Operator=transpose  SaturateOnIntegerOverflow=on
  Product : Product  Inputs=3  Multiplication=Matrix(*)
  tag scope: Manip3KineticEnergy=global
  wires:
  dx/1 -> Product/3, Math Function/1
  Math Function/1 -> Product/1
  Constant/1 -> Product/2
  Product/1 -> [Manip3KineticEnergy]

== system DIPCRT/Manipulator Springs/Spring 3/Spring Energy ==
  deltax : Inport
  Constant : Constant  Value=blkdiag(0.5*ks*eye(3),2*kappas*eye(3))
  Math Function : Math  Operator=transpose  SaturateOnIntegerOverflow=on
  Product : Product  Inputs=3  Multiplication=Matrix(*)
  tag scope: Manip3SpringEnergy=global
  wires:
  deltax/1 -> Product/3, Math Function/1
  Math Function/1 -> Product/1
  Constant/1 -> Product/2
  Product/1 -> [Manip3SpringEnergy]

== system DIPCRT/Manipulator Springs/Spring 4/Angular Velocity to Quaternion ==
  omega_o : Inport
  Constant : Constant  Value=0
  Gain : Gain  Gain=0.5
  Integrator : Integrator  InitialCondition=[1; 0; 0; 0]
  Mux : Mux  Inputs=2
  Quaternion Multiplication : aerolibutil/Quaternion Multiplication
  Quaternion Normalize : aerolibutil/Quaternion Normalize
  q_o : Outport
  wires:
  omega_o/1 -> Gain/1
  Gain/1 -> Mux/2
  Constant/1 -> Mux/1
  Quaternion Multiplication/1 -> Integrator/1
  Integrator/1 -> Quaternion Normalize/1
  Mux/1 -> Quaternion Multiplication/1
  Quaternion Normalize/1 -> Quaternion Multiplication/2, q_o/1

== system DIPCRT/Manipulator Springs/Spring 4/Kinetic energy ==
  dx : Inport
  Constant : Constant  Value=blkdiag(0.5*m4*eye(3),0.5*j4*eye(3))
  Math Function : Math  Operator=transpose  SaturateOnIntegerOverflow=on
  Product : Product  Inputs=3  Multiplication=Matrix(*)
  tag scope: Manip4KineticEnergy=global
  wires:
  dx/1 -> Product/3, Math Function/1
  Math Function/1 -> Product/1
  Constant/1 -> Product/2
  Product/1 -> [Manip4KineticEnergy]

== system DIPCRT/Manipulator Springs/Spring 4/Spring Energy ==
  deltax : Inport
  Constant : Constant  Value=blkdiag(0.5*ks*eye(3),2*kappas*eye(3))
  Math Function : Math  Operator=transpose  SaturateOnIntegerOverflow=on
  Product : Product  Inputs=3  Multiplication=Matrix(*)
  tag scope: Manip4SpringEnergy=global
  wires:
  deltax/1 -> Product/3, Math Function/1
  Math Function/1 -> Product/1
  Constant/1 -> Product/2
  Product/1 -> [Manip4SpringEnergy]

== matlab function DIPCRT/Manipulator Springs/Spring 1/Manipualtor pose in world frame ==
  data: pb input; qb input size=4; pb1 output; rv parameter; qb1 output
function [pb1,qb1]= manipulatorpose(pb,qb,rv)

pb1 = pb + quatrot(qb,rv(1:3));
qb1 = qb;

== matlab function DIPCRT/Manipulator Springs/Spring 2/Manipualtor pose in world frame ==
  data: pb input; qb input size=4; pb2 output; rv parameter; qb2 output
function [pb2,qb2]= manipulatorpose(pb,qb,rv)

pb2 = pb + quatrot(qb,rv(4:6));
qb2 = qb;

== matlab function DIPCRT/Manipulator Springs/Spring 3/Manipualtor pose in world frame ==
  data: pb input; qb input size=4; pb3 output; rv parameter; qb3 output
function [pb3,qb3]= manipulatorpose(pb,qb,rv)

pb3 = pb + quatrot(qb,rv(7:9));
qb3 = qb;

== matlab function DIPCRT/Manipulator Springs/Spring 4/Manipualtor pose in world frame ==
  data: pb input; qb input size=4; pb4 output; rv parameter; qb4 output
function [pb4,qb4]= manipulatorpose(pb,qb,rv)

pb4 = pb + quatrot(qb,rv(10:12));
qb4 = qb;
